simulink model "varbounds_sim"  (Simulink 5.0)
settings: Solver=ode45  StartTime=0.0  StopTime=Tstop  RelTol=1e-3
values from neighbouring files (symbols this model uses):
  C1 = lincon(model,'track',cost,interval,limits)    [example1.m]    (also in example3.m; timevarying1.m = lincon(themodel,'track',cost,interval,limits); varbounds.m = kalmdesign(C1,Qn,Rn,ymeasured))
  Tstop = 80*Ts    (= 4)    [afti16.m]    (also in bmdp02.m; dcmotor.m = 20; doubleint.m = 40; doubleintexp.m = 40)
libraries: simulink x2, cstblocks x1, hyblib x1
settings Model: LastModifiedBy=Alberto Bemporad  ExtModeTrigMode=oneshot  ExtModeArmWhenConnect=off  LimitDataPoints=off  BooleanDataType=off

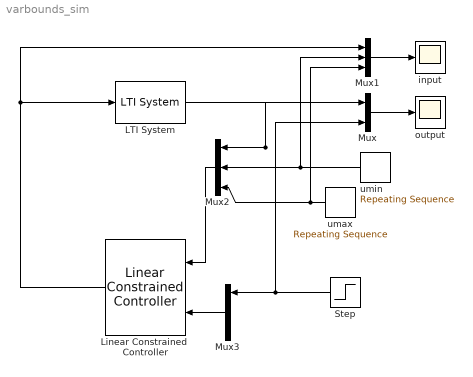
== system varbounds_sim ==
  LTI System : cstblocks/LTI System  sys=sys  IC=0
  Linear Constrained  Controller : hyblib/Linear Constrained  Controller  Orientation=left  C=C1  xhat0=x0  u1=0
  Mux : Mux  Inputs=2
  Mux1 : Mux  Inputs=3
  Mux2 : Mux  Orientation=left  Inputs=3
  Mux3 : Mux  Orientation=left  Inputs=3
  Step : Step  Orientation=left  Time=0  Before=1  SampleTime=0
  input : Scope
      settings: TimeRange=20  YMin=-2  YMax=4
  output : Scope
      settings: TimeRange=20  YMin=0  YMax=1.5
  umax : simulink/Sources/Repeating Sequence  Orientation=left  rep_seq_t=[0 1 6 Tstop]  rep_seq_y=[3 2 4 3]
  umin : simulink/Sources/Repeating Sequence  Orientation=left  rep_seq_t=[0 2 4 Tstop]  rep_seq_y=[-1 -2 -1 -2]
  wires:
  LTI System/1 -> Mux/1, Mux2/1
  Mux/1 -> output/1
  Linear Constrained  Controller/1 -> LTI System/1, Mux1/1
  Step/1 -> Mux/2, Mux3/1
  Mux1/1 -> input/1
  Mux2/1 -> Linear Constrained  Controller/1
  umin/1 -> Mux2/2, Mux1/2
  umax/1 -> Mux2/3, Mux1/3
  Mux3/1 -> Linear Constrained  Controller/2
